simulink model "complex_sub"  (R2013b)
settings: Solver=ode45  StartTime=0.0  StopTime=10.0  RelTol=1e-3
libraries: casper_library_misc x3, xbsIndex_r4 x2
settings Model: Creator=root  LastModifiedBy=root

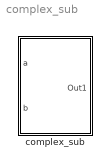
== system complex_sub ==
  complex_sub : Subsystem  mask(complex_sub){a_bitsize=10, b_bitsize=10, latency=0}
      mask init:
      | complex_sub_init(gcb, ...
      |             'a_bitsize', a_bitsize, ...
      |             'b_bitsize', b_bitsize, ...
      |             'latency', latency);
      settings: AttributesFormatString=latency=0

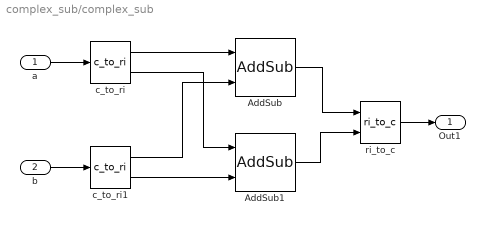
== system complex_sub/complex_sub ==
  "a " : Inport
  b : Inport  Port=2
  AddSub : xbsIndex_r4/AddSub  mode=Subtraction  use_carryin=off  use_carryout=off  en=off  latency=latency  precision=Full  arith_type=Unsigned  n_bits=16  bin_pt=14  quantization=Truncate  overflow=Wrap  dbl_ovrd=off  use_behavioral_HDL=off  hw_selection=Fabric  pipelined=off  block_type=addsub
  AddSub1 : xbsIndex_r4/AddSub  mode=Subtraction  use_carryin=off  use_carryout=off  en=off  latency=latency  precision=Full  arith_type=Unsigned  n_bits=16  bin_pt=14  quantization=Truncate  overflow=Wrap  dbl_ovrd=off  use_behavioral_HDL=off  hw_selection=Fabric  pipelined=off  block_type=addsub
  c_to_ri : casper_library_misc/c_to_ri  n_bits=a_bitsize  bin_pt=a_bitsize-1
      settings: AttributesFormatString=10_9 r/i
  c_to_ri1 : casper_library_misc/c_to_ri  n_bits=b_bitsize  bin_pt=b_bitsize-1
      settings: AttributesFormatString=0_-1 r/i
  ri_to_c : casper_library_misc/ri_to_c
  Out1 : Outport
  wires:
  "a "/1 -> c_to_ri/1
  b/1 -> c_to_ri1/1
  c_to_ri/1 -> AddSub/1
  c_to_ri1/1 -> AddSub/2
  c_to_ri/2 -> AddSub1/1
  c_to_ri1/2 -> AddSub1/2
  AddSub/1 -> ri_to_c/1
  AddSub1/1 -> ri_to_c/2
  ri_to_c/1 -> Out1/1
